simulink model "hw6_system"  (R2022a)
settings: Solver=VariableStepAuto  StartTime=0.0  StopTime=10.0  RelTol=1e-3
values from neighbouring files (symbols this model uses):
  B = 0.5    [hw6.m]    (also in hw6_q2.m; hw6_q3.m; hw6_q4.m; hw6_q5.m)
  J = 2    [hw6.m]    (also in hw6_q2.m; hw6_q3.m; hw6_q4.m; hw6_q5.m)
  K_d = 8    [hw6.m]    (also in hw6_q2.m = 7.5; hw6_q3.m = 7.5; hw6_q4.m; hw6_q5.m)
  K_p = 11.55    [hw6.m]    (also in hw6_q2.m = 8; hw6_q3.m = 8; hw6_q4.m = 11; hw6_q5.m = 11)
settings Model: Creator=arjan  LastModifiedBy=arjan

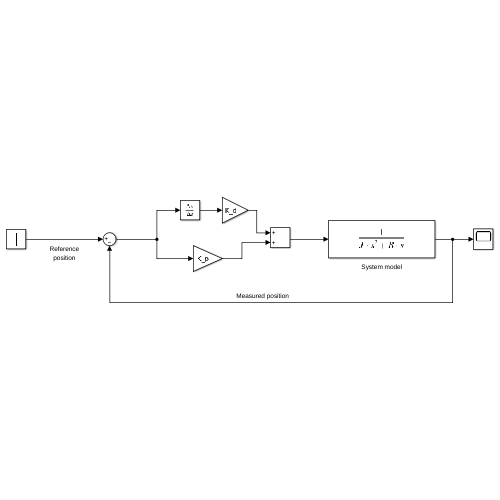
[thumbnail: Simulink's stored preview of the top-level diagram]
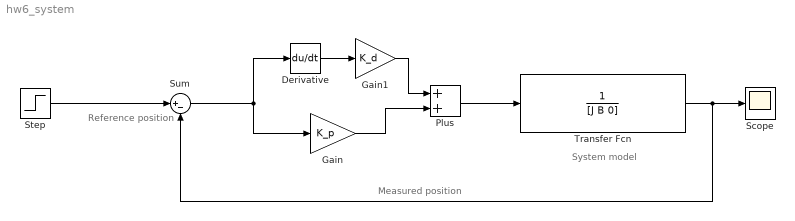
== system hw6_system ==
  note: Reference
      | position
  note: Measured position
  note: System model
  Derivative : Derivative
  Gain : Gain  Gain=K_p
  Gain1 : Gain  Gain=K_d
  Plus : Sum
  Scope : Scope
  Step : Step  SampleTime=0
  Sum : Sum  Inputs=|+-
  Transfer Fcn : TransferFcn  Denominator=[J B 0]
  wires:
  Sum/1 -> Gain/1, Derivative/1
  Transfer Fcn/1 -> Sum/2, Scope/1
  Derivative/1 -> Gain1/1
  Plus/1 -> Transfer Fcn/1
  Gain1/1 -> Plus/1
  Gain/1 -> Plus/2
  Step/1 -> Sum/1
